simulink model "sim_b"  (R2019a)
settings: Solver=FixedStepAuto  StartTime=0.0  StopTime=3.0  FixedStep=0.01  RelTol=1e-3
values from neighbouring files (symbols this model uses):
  b = 0.5    [zero_cancelation.m]
  ti = kp / ki    [zero_cancelation.m]
undefined symbols (not defined in the file or in its folder): k, kp, tau1
settings Model: Creator=jessicaliporace  LastModifiedBy=jessicaliporace

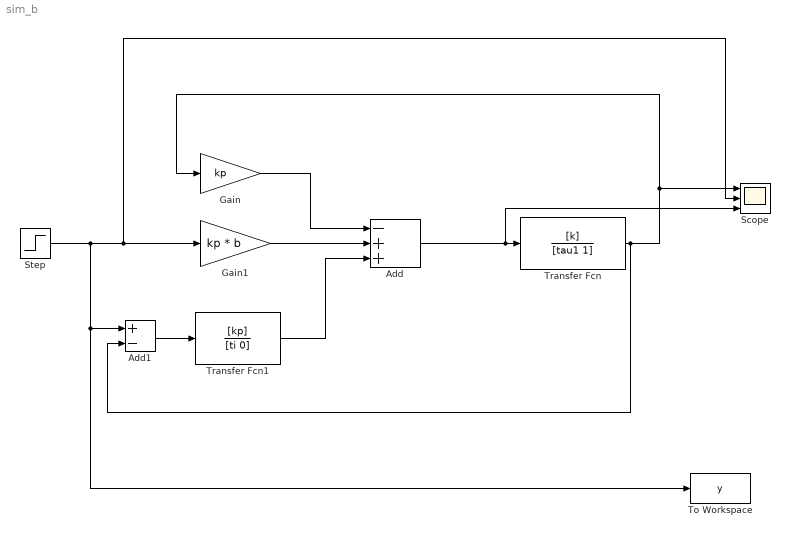
== system sim_b ==
  Add : Sum  Inputs=-++
  Add1 : Sum  Inputs=+-
  Gain : Gain  Gain=kp
  Gain1 : Gain  Gain=kp * b
  Scope : Scope  NumInputPorts=3
  Step : Step  SampleTime=0
  To Workspace : ToWorkspace  VariableName=y  SampleTime=0.01
  Transfer Fcn : TransferFcn  Numerator=[k]  Denominator=[tau1 1]
  Transfer Fcn1 : TransferFcn  Numerator=[kp]  Denominator=[ti 0]
  wires:
  Transfer Fcn/1 -> Add1/2, Gain/1, Scope/1
  Step/1 -> Add1/1, To Workspace/1, Scope/2, Gain1/1
  Add/1 -> Scope/3, Transfer Fcn/1
  Gain1/1 -> Add/2
  Gain/1 -> Add/1
  Transfer Fcn1/1 -> Add/3
  Add1/1 -> Transfer Fcn1/1
